simulink model "PIDController"  (R2019b)
settings: Solver=VariableStepAuto  StartTime=0.0  StopTime=10.0  RelTol=1e-3
undefined symbols (not defined in the file or in its folder): b, J, Ke, Kt, L, R
settings Model: DataDictionary=Data_Dict.sldd  Creator=ip  LastModifiedBy=ip

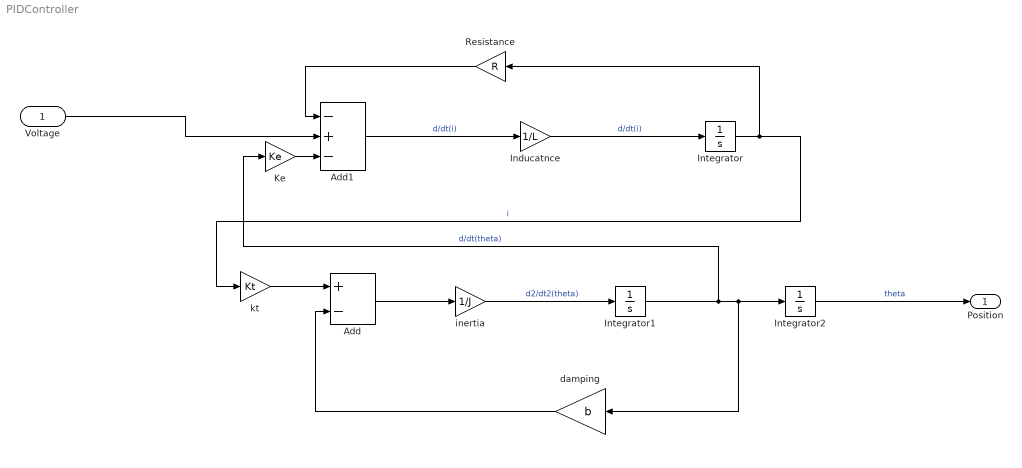
== system PIDController ==
  Voltage : Inport
  Add : Sum  Inputs=+-
  Add1 : Sum  Inputs=-+-
  Inducatnce : Gain  Gain=1/L
  Integrator : Integrator
  Integrator1 : Integrator
  Integrator2 : Integrator
  Ke : Gain  Gain=Ke
  Resistance : Gain  Gain=R
  damping : Gain  Gain=b
  inertia : Gain  Gain=1/J
  kt : Gain  Gain=Kt
  Position : Outport
  wires:
  Integrator2/1 -> Position/1  "theta"
  Resistance/1 -> Add1/1
  Add1/1 -> Inducatnce/1  "d/dt(i)"
  kt/1 -> Add/1
  Inducatnce/1 -> Integrator/1  "d/dt(i)"
  Integrator1/1 -> Ke/1, damping/1, Integrator2/1  "d/dt(theta)"
  damping/1 -> Add/2
  Ke/1 -> Add1/3
  Voltage/1 -> Add1/2
  inertia/1 -> Integrator1/1  "d2/dt2(theta)"
  Add/1 -> inertia/1
  Integrator/1 -> kt/1, Resistance/1  "i"
